simulink model "se3"  (R2020a)
settings: Solver=FixedStepAuto  StartTime=0.0  StopTime=100  FixedStep=0.005  RelTol=1e-3
settings Model: Creator=isxie  LastModifiedBy=isxie

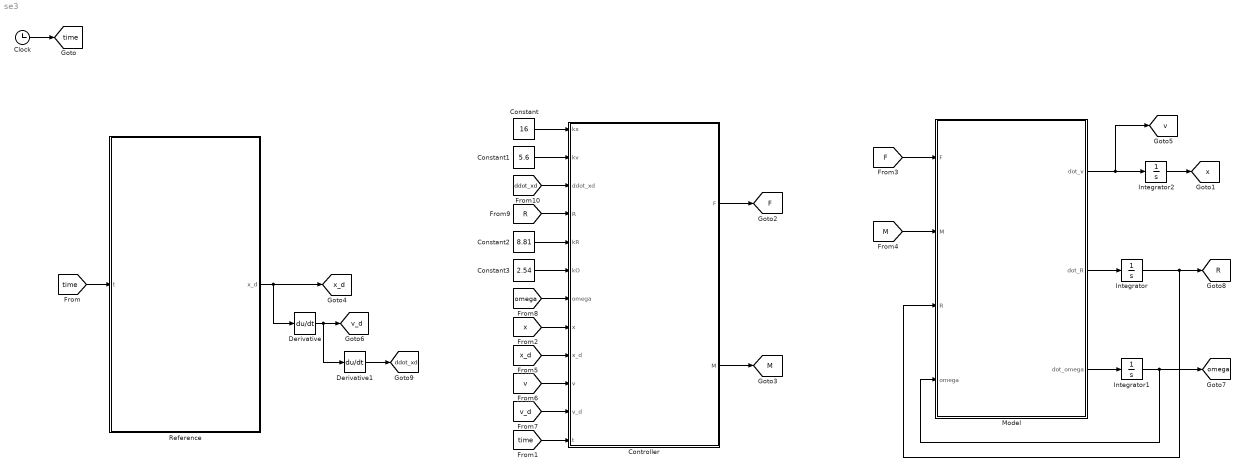
== system se3 ==
  Clock : Clock
  Constant : Constant  Value=16
  Constant1 : Constant  Value=5.6
  Constant2 : Constant  Value=8.81
  Constant3 : Constant  Value=2.54
  Controller : MATLAB Function  TreatAsAtomicUnit=on
  Derivative : Derivative
  Derivative1 : Derivative
  Integrator : Integrator  InitialCondition=[1,0,0;0,1,0;0,0,1]
  Integrator1 : Integrator  InitialCondition=[0;0;0]
  Integrator2 : Integrator  InitialCondition=[0;0;0]
  Model : MATLAB Function  TreatAsAtomicUnit=on
  Reference : MATLAB Function  TreatAsAtomicUnit=on
  tag scope: F=global, M=global, R=global, ddot_xd=global, omega=global, time=global, v=global, v_d=global, x=global, x_d=global
  wires:
  Clock/1 -> [time]
  [time] -> Reference/1(t)
  [time] -> Controller/12(t)
  Model/2(dot_R) -> Integrator/1
  Model/3(dot_omega) -> Integrator1/1
  Integrator1/1 -> Model/4(omega), [omega]
  Integrator/1 -> [R], Model/3(R)
  Model/1(dot_v) -> [v], Integrator2/1
  Integrator2/1 -> [x]
  [x] -> Controller/8(x)
  Controller/1(F) -> [F]
  Controller/2(M) -> [M]
  [M] -> Model/2(M)
  [F] -> Model/1(F)
  Reference/1(x_d) -> Derivative/1, [x_d]
  [x_d] -> Controller/9(x_d)
  [v] -> Controller/10(v)
  Derivative/1 -> Derivative1/1, [v_d]
  [v_d] -> Controller/11(v_d)
  Constant/1 -> Controller/1(kx)
  Constant1/1 -> Controller/2(kv)
  Constant2/1 -> Controller/5(kR)
  Constant3/1 -> Controller/6(kO)
  [omega] -> Controller/7(omega)
  [R] -> Controller/4(R)
  Derivative1/1 -> [ddot_xd]
  [ddot_xd] -> Controller/3(ddot_xd)

== matlab function se3/Controller ==
  data: kx input; kv input; ddot_xd input; R input; kR input; kO input; omega input; F output; x input; x_d input; v input; v_d input; M output; t input
function [F,M] = fcn(kx,kv,ddot_xd,R,kR,kO,omega,x,x_d,v,v_d,t)

m = 4.34; g = 9.8; J = diag([0.082;0.0845;0.1377]); e3 = [0;0;1];

ex = x-x_d; ev = v-v_d; 

b1_d = [cos(pi*t);sin(pi*t);0];
b3_d = -(-kx*ex-kv*ev-m*g*e3+m*ddot_xd)/(norm(-kx*ex-kv*ev-m*g*e3+m*ddot_xd));
b2_d = (cross(b3_d,b1_d))/norm(cross(b3_d,b1_d));
Rd = [cross(b2_d,b3_d),b2_d,b3_d];
dot_Rd = diff(Rd);
omega_d_mid = Rd'*dot_Rd;
omega_d = [omega_d_mid(3,2);omega_d_mid(1,3);omega_d_mid(2,1)];
dot_omega_d = diff(omega_d);

eR_mid = 1/2*(Rd'*R-R'*Rd);
eR = [eR_mid(3,2);eR_mid(1,3);eR_mid(2,1)];
eO = omega - R'*Rd*omega_d;

F1 = -(-kx*ex-kv*ev-m*g*e3+m*ddot_xd);
F2 = R*e3;
sk_omega = [0,-omega(3),omega(2);omega(3),0,-omega(1);-omega(2),omega(1),0];
F = dot(F1,F2);
M = -kR*eR-kO*eO+cross(omega,(J*omega))-J*(sk_omega*R'*Rd*omega_d-R'*Rd*dot_omega_d);

== matlab function se3/Reference ==
  data: t input; x_d output
function x_d  = fcn(t)

x = 0.4*t;
y = 0.4*sin(pi*t);
z = 0.4*cos(pi*t);
x_d = [x;y;z];

== matlab function se3/Model ==
  data: dot_v output; dot_R output; F input; M input; R input; omega input; dot_omega output
function [dot_v,dot_R,dot_omega] = fcn(F,M,R,omega)

J = diag([0.082;0.0845;0.1377]); m = 4.34; e3 = [0;0;1]; g = 9.8;

sk = [0,-omega(3),omega(2);omega(3),0,-omega(1);-omega(2),omega(1),0];
dot_v = g*e3-1/m*F*R*e3;
dot_R = R*sk;
dot_omega = inv(J)*(-sk*(J*omega)+M);
